simulink model "time_domain_array_sinusoidal_input"  (R2016a)
settings: Solver=ode15s  StartTime=0.0  StopTime=10.0  RelTol=1e-9
values from neighbouring files (symbols this model uses):
  excitation_frequency = omega(omega_num)    [td_v_WAMIT_fd_comparison.m]
  inv_reduced_mass_matrix = inv(reduced_mass_matrix)    [create_td_WEC_array_model.m]
  Mod_X_i = zeros(1,num_modes)    [td_v_WAMIT_fd_comparison.m]
  Pha_X_i = pi_over_180*              excite_forces(offset+1:offset+num_modes,5)    [td_v_WAMIT_fd_comparison.m]
  reduced_damping_matrix = zeros(num_dofs,num_dofs)    [create_td_WEC_array_model.m]
  reduced_stiffness_matrix = zeros(num_dofs,num_dofs)    [create_td_WEC_array_model.m]
  sys = ss(H)    [create_td_WEC_array_model.m]    (also in get_TF.m = tf(TFnum,TFden))
settings Model: Creator=dforehan  LastModifiedBy=dforehan
settings DataIOCC: LimitDataPoints=on  SaveFormat=Array  SignalLoggingSaveFormat=ModelDataLogs
settings OptimizationCC: ExpressionDepthLimit=2147483647  InitFltsAndDblsToZero=on
settings DebuggingCC: UnderspecifiedInitializationDetection=Classic  MergeDetectMultiDrivingBlocksExec=none  SolverPrmCheckMsg=warning  FcnCallInpInsideContextMsg=UseLocalSettings  StateNameClashWarn=warning  StrictBusMsg=Warning
settings HardwareCC: ProdBitPerPointer=32  ProdLargestAtomicFloat=None  ProdIntDivRoundTo=Undefined  ProdEndianess=Unspecified  ProdWordSize=32  ProdHWDeviceType=32-bit Generic
settings ModelReferenceCC: PropagateSignalLabelsOutOfModel=off
settings GRTTargetCC: GeneratePreprocessorConditionals=Use local settings  CombineOutputUpdateFcns=off  GRTInterface=on
settings ConfigComp: CovModelRefEnable=Off

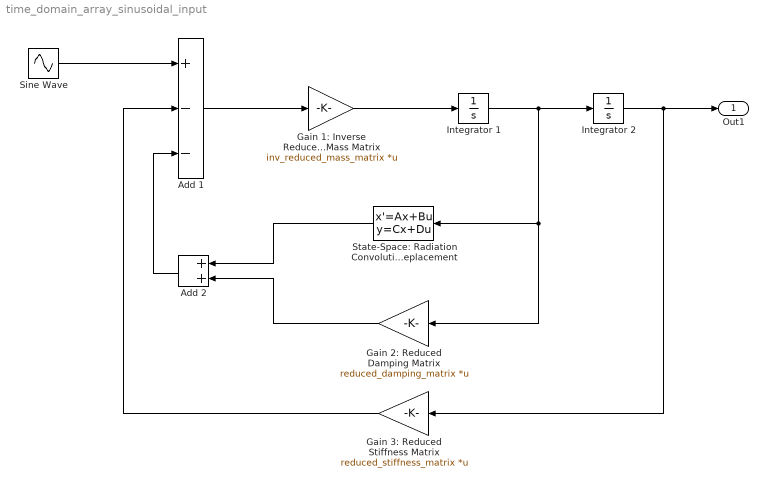
== system time_domain_array_sinusoidal_input ==
  Add 1 : Sum  Inputs=+--
  Add 2 : Sum
  Gain 1: Inverse Reduced Mass Matrix : Gain  Gain=inv_reduced_mass_matrix  Multiplication=Matrix(K*u)
  Gain 2: Reduced Damping Matrix : Gain  Gain=reduced_damping_matrix  Multiplication=Matrix(K*u)
  Gain 3: Reduced Stiffness Matrix : Gain  Gain=reduced_stiffness_matrix  Multiplication=Matrix(K*u)
  Integrator 1 : Integrator
  Integrator 2 : Integrator
  Sine Wave : Sin  Amplitude=Mod_X_i  Frequency=excitation_frequency  Phase=Pha_X_i  SampleTime=0
  State-Space: Radiation Convolution Replacement : StateSpace  A=sys.a  B=sys.b  C=sys.c  D=sys.d  X0=0
  Out1 : Outport
  wires:
  Sine Wave/1 -> Add 1/1
  Add 1/1 -> Gain 1: Inverse Reduced Mass Matrix/1
  Gain 1: Inverse Reduced Mass Matrix/1 -> Integrator 1/1
  Integrator 2/1 -> Out1/1, Gain 3: Reduced Stiffness Matrix/1
  Integrator 1/1 -> Integrator 2/1, Gain 2: Reduced Damping Matrix/1, State-Space: Radiation Convolution Replacement/1
  State-Space: Radiation Convolution Replacement/1 -> Add 2/1
  Gain 2: Reduced Damping Matrix/1 -> Add 2/2
  Gain 3: Reduced Stiffness Matrix/1 -> Add 1/2
  Add 2/1 -> Add 1/3
